simulink model "physical_model"  (R2016b)
settings: Solver=VariableStepAuto  StartTime=0.0  StopTime=3000  FixedStep=1  RelTol=1e-3  AbsTol=1e-6
model workspace (MATLAB code in the model file):
  | % load initial conditions and physical properties from file
  | 
  | %sldemo_househeat_data
  | househeat_data_szakdoga
  | 
  | addpath('subsystems')
  | 
  | %disp('adding models...')
  | load('subsystems/mpc_floor_radiator.mat')
  | %disp('done.')
values from neighbouring files (symbols this model uses):
  A_heater = 3.5    [househeat_data_szakdoga.m]
  c = 1005.4    [househeat_data_szakdoga.m]
  h_heater = 11    [househeat_data_szakdoga.m]
  M = (lenHouse*widHouse*htHouse+tan(pitRoof)*widHouse*lenHouse)*densAir    [househeat_data_szakdoga.m]    (also in thesismpcmiso.m = A1\L)
  Req = RWall*RWindow/(RWall + RWindow)    [househeat_data_szakdoga.m]
  supp_water_initial_temp = 0    [househeat_data_szakdoga.m]
  TinHeatK = 273    [househeat_data_szakdoga.m]
  TinIC = 0    [househeat_data_szakdoga.m]
undefined symbols (not defined in the file or in its folder): timeUnit_1hour, timeUnit_1min, timeUnit_1week
libraries: fl_lib x37, nesl_utility x14, simulink x3, instrumentlib x3, xpcrtudplib x3, slident x1, mpclib x1
Description:
  | Thermal Model of a House
  | 
  | This demo illustrates how you can use Simulink(R) to create the thermal model of
  | a house. This system models the outdoor environment, the thermal
  | characteristics of the house, and the house heating system.
  | 
  | The sldemo_househeat_data.m file initializes data in the model workspace.
  | To make changes, you can edit the model workspace directly or edit the MATLAB(R) file
  | and re-load the model workspace.
  | 
  | To view the model workspace, select View > Model Explorer
  | from the Simulink editor.
  | 
  | Note: Time is given in units of hours
settings Model: PauseTimes=10  ExtModeTrigMode=oneshot  ExtModeArmWhenConnect=off  ExtModeAutoUpdateStatusClock=off  Creator=The MathWorks, Inc.  LastModifiedBy=gylaszlo
settings DataIOCC: ExternalInput=[]  InitialState=[]  SaveFormat=StructureWithTime  SaveOutput=off  SaveTime=off  SignalLoggingName=sldemo_househeat_output
settings OptimizationCC: BlockReduction=off  BooleanDataType=off  ExpressionDepthLimit=2147483647  InitFltsAndDblsToZero=on  LifeSpan=inf  BufferReusableBoundary=off
settings DebuggingCC: SaveWithParameterizedLinksMsg=none  UnderspecifiedInitializationDetection=Classic  MergeDetectMultiDrivingBlocksExec=none  SignalResolutionControl=TryResolveAllWithWarning  MultiTaskDSMMsg=warning  MultiTaskCondExecSysMsg=none  IntegerOverflowMsg=none  FcnCallInpInsideContextMsg=warning  BusObjectLabelMismatch=none  StateNameClashWarn=warning  SFUnexpectedBacktrackingDiag=warning  SFNoUnconditionalDefaultTransitionDiag=warning  SFExecutionAtInitializationDiag=none  IntegerSaturationMsg=none
settings HardwareCC: ProdBitPerPointer=32  ProdBitPerSizeT=32  ProdBitPerPtrDiffT=32  ProdLargestAtomicFloat=None  ProdIntDivRoundTo=Undefined  ProdEndianess=Unspecified  ProdWordSize=32  ProdHWDeviceType=32-bit Generic  TargetUnknown=on
settings ModelReferenceCC: PropagateSignalLabelsOutOfModel=off
settings GRTTargetCC: TargetFcnLib=ansi_tfl_tmw.mat  TargetLangStandard=C89/C90 (ANSI)  GeneratePreprocessorConditionals=Disable all  CombineOutputUpdateFcns=off  GRTInterface=on
settings ConfigComp: CovMetricSettings=dw  CovHtmlReporting=on  CovSaveCumulativeToWorkspaceVar=on  CovSaveSingleToWorkspaceVar=on  CovExternalEMLEnable=off

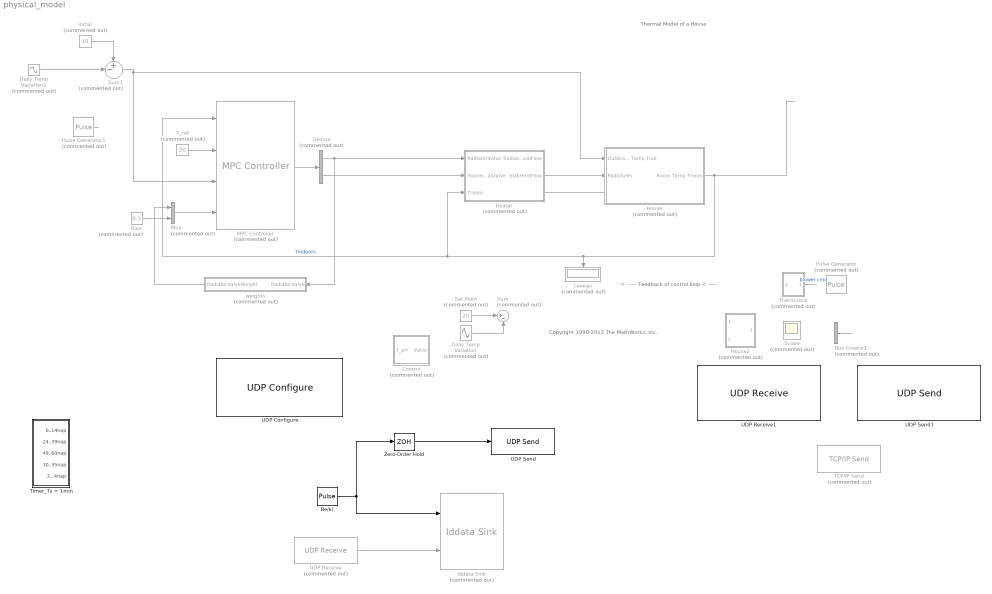
== system physical_model ==
  note: < ------ Feedback of control loop < ------
  note: Thermal Model of a House
  note: Copyright 1990-2012 The MathWorks, Inc.
  Be/ki : DiscretePulseGenerator  PulseType=Time based  Amplitude=100  Period=120  PulseWidth=50
  Bus Creator1 : BusCreator  Commented=on  Inputs=2
  Control : Subsystem  Commented=on
  Daily Temp Variation : Sin  Commented=on  Amplitude=5  Frequency=3.14*2/3600/24  Phase=3.14/2  SampleTime=0
  Daily Temp Variation1 : Sin  Commented=on  Amplitude=5  Frequency=3.14*2/3600/24  Phase=3.14/2  SampleTime=0
  Demux : Demux  Commented=on  Outputs=2
  Heater : Subsystem  Commented=on
  House : Subsystem  Commented=on
  House2 : Subsystem  Commented=on
      mask Display: image(fullfile(matlabroot,'toolbox','simulink','simdemos','simgeneral','images','HouseHeatHousePix.svg'))
  Iddata Sink : slident/Iddata Sink  Commented=on  datasetname=meres  Ts=10  isu=off  isy=off
  Levego : Display  Commented=on
  MPC Controller : mpclib/MPC Controller  Commented=on  SCDEnableBlockLinearizationSpecification=on  mpcobj=mpc_floor_radiator  is_multiple=0  enable_value=0  return_u0=off  ref_from_ws=off  ref_signal_name=[]  ref_preview=off  md_from_ws=off  md_signal_name=[]  md_preview=off  from_project=off  project_file=MPCtask.mat  md_inport=on  mv_inport=off  cost_outport=off  return_sequence=off  return_qpstatus=off  return_state=off  state_inport=off  lims_inport=off  ywt_inport=off  is_designfromscratch=0  uwt_inport=on  duwt_inport=off  rhoeps_inport=off  uref_inport=off  n_ts=300  n_mv=2  n_md=1  n_ud=0  n_mo=1  n_uo=0  BlockDataType=double  SampleTimeInherited=off  switch_inport=off
  Mux : Mux  Commented=on  Inputs=2
  Pulse Generator : DiscretePulseGenerator  Commented=on  PulseType=Time based  Period=3600*24*4  PulseWidth=50
  Pulse Generator1 : DiscretePulseGenerator  Commented=on  PulseType=Time based  Amplitude=15  Period=3600*24*4  PulseWidth=50
  Scope : Scope  Commented=on
  Set Point : Constant  Commented=on  Value=20
  Sum : Sum  Commented=on  Inputs=+-|  SaturateOnIntegerOverflow=on  InputSameDT=on  OutDataTypeStr=Inherit: Same as first input
  Sum1 : Sum  Commented=on  Inputs=+-|  SaturateOnIntegerOverflow=on  InputSameDT=on  OutDataTypeStr=Inherit: Same as first input
  TCP/IP Send : instrumentlib/TCP//IP Send  Commented=on  Host=192.168.0.108  Port=9090  EnableBlockingMode=on  Timeout=10  ByteOrder=BigEndian
  T_ref : Constant  Commented=on  Value=20
  Thermostat : Subsystem  Commented=on
      mask Display: image(fullfile(matlabroot,'toolbox','simulink','simdemos','simgeneral','images','HouseHeatThermostatPix.svg'))
  Timer_Ts = 1min : Subsystem
  UDP Configure : xpcrtudplib/UDP Configure  Priority=-1  IpAddress=192.168.0.136  SubnetMask=255.255.255.0  Gateway=192.168.0.1  PciBus=2  PciSlot=0  ID=1  tune=0
  UDP Receive : instrumentlib/UDP Receive  Commented=on  Port=9090  LocalPort=-1  DataSize=[1 1]  EnableBlockingMode=on  Timeout=10  SampleTime=0.01  DataType=uint8  ByteOrder=BigEndian
  UDP Receive1 : xpcrtudplib/UDP Receive  ipAddressVal=Use host-target connection  localPort=8001  rcvWidth=16  rcvFmAny=on  fmAddress=0.0.0.0  sampleTime=-1
  UDP Send : instrumentlib/UDP Send  Host=192.168.0.108  Port=9090  LocalPort=-1  EnableBlockingMode=on  ByteOrder=BigEndian
  UDP Send1 : xpcrtudplib/UDP Send  ipAddressVal=Use host-target connection  localPort=9090  toAddress=168.192.0.108  toPort=9090  sampleTime=-1
  Zero-Order Hold : ZeroOrderHold  SampleTime=10
  floor : Constant  Commented=on  Value=0.3
  initial : Constant  Commented=on  Value=10
  weights : Subsystem  Commented=on
  wires:
  ? -> Control/1(T_err)  "Terr"
  House/1(Room Temp Troom) -> Heater/3(Troom), MPC Controller/1, Levego/1  "Tindoors"
  Set Point/1 -> Sum/1
  Thermostat/1(Blower switch) -> ?  "blower cmd"
  Bus Creator1/1 -> ?
  Sum1/1 -> MPC Controller/3, House/1(Outdoor Temp Tout)
  Daily Temp Variation/1 -> Sum/2
  T_ref/1 -> MPC Controller/2
  Heater/2(SlabHeatFlow) -> House/2(Padlofutes)
  Daily Temp Variation1/1 -> Sum1/2
  initial/1 -> Sum1/1
  MPC Controller/1 -> Demux/1
  Demux/2 -> Heater/2(FloorHeatValve)
  Demux/1 -> weights/1(RadiatorValve), Heater/1(RadiatorValve)
  Pulse Generator1/1 -> ?
  weights/1(RadiatorValveWeight) -> Mux/1
  floor/1 -> Mux/2
  Mux/1 -> MPC Controller/4
  UDP Receive/1 -> Iddata Sink/2
  Be/ki/1 -> Zero-Order Hold/1, Iddata Sink/1
  Zero-Order Hold/1 -> UDP Send/1
  connections:
  House/LConn1 -- Heater/RConn1

== system physical_model/Control ==
  note: valve opening rate
  T_err : Inport
  PID Controller : simulink/Continuous/PID Controller  Controller=PI  TimeDomain=Continuous-time  SampleTime=-1  IntegratorMethod=Forward Euler  FilterMethod=Forward Euler  Form=Parallel  UseFilter=on  ControllerParametersSource=internal  P=0.09  I=9.95e-07  D=0  N=100  InitialConditionSource=internal  InitialConditionForIntegrator=0  InitialConditionForFilter=0  ExternalReset=none  LimitOutput=on  UpperSaturationLimit=1  LowerSaturationLimit=0  LinearizeAsGain=on  AntiWindupMode=none  Kb=1  TrackingMode=off  Kt=1  PParamMin=[]  PParamMax=[]  IParamMin=[]  IParamMax=[]  DParamMin=[]  DParamMax=[]  NParamMin=[]  NParamMax=[]  KbParamMin=[]  KbParamMax=[]  KtParamMin=[]  KtParamMax=[]  POutMin=[]  POutMax=[]  IOutMin=[]  IOutMax=[]  DOutMin=[]  DOutMax=[]  NOutMin=[]  NOutMax=[]  KbOutMin=[]  KbOutMax=[]  KtOutMin=[]  KtOutMax=[]  IntegratorOutMin=[]  IntegratorOutMax=[]  FilterOutMin=[]  FilterOutMax=[]  SumOutMin=[]  SumOutMax=[]  SumI1OutMin=[]  SumI1OutMax=[]  SumI2OutMin=[]  SumI2OutMax=[]  SumI3OutMin=[]  SumI3OutMax=[]  SumDOutMin=[]  SumDOutMax=[]  SaturationOutMin=[]  SaturationOutMax=[]  IntegratorContinuousStateAttributes=''  IntegratorStateMustResolveToSignalObject=off  IntegratorRTWStateStorageClass=Auto  FilterContinuousStateAttributes=''  FilterStateMustResolveToSignalObject=off  FilterRTWStateStorageClass=Auto  DifferentiatorICPrevScaledInput=0  DifferentiatorOutMin=[]  DifferentiatorOutMax=[]
  Valve : Outport
  wires:
  T_err/1 -> PID Controller/1
  PID Controller/1 -> Valve/1

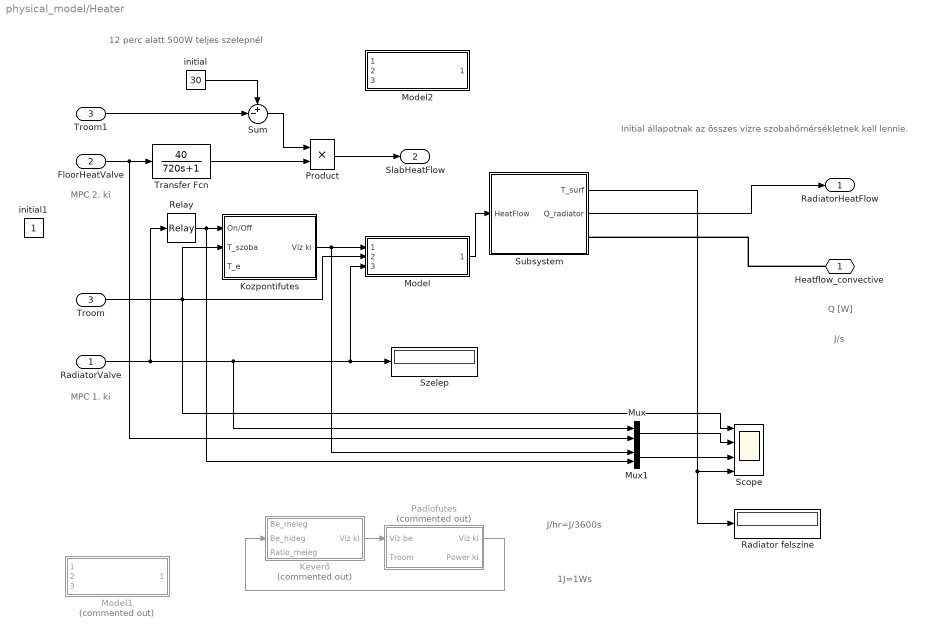
== system physical_model/Heater ==
  note: MPC 1. ki
  note: 12 perc alatt 500W teljes szelepnél
  note: Initial állapotnak az összes vízre szobahőmérsékletnek kell lennie.
  note: J/s
  note: 1J=1Ws
  note: J/hr=J/3600s
  note: Q [W]
  note: MPC 2. ki
  RadiatorValve : Inport
  FloorHeatValve : Inport  Port=2
  Troom : Inport  Port=3
  Keverő : Subsystem  Commented=on
  Kozpontifutes : Subsystem
  Model : ModelReference  ModelNameDialog=Radiator  SimulationMode=Normal  ModelReferenceVersion=1.21
  Model1 : ModelReference  Commented=on  ModelNameDialog=Radiator  SimulationMode=Normal  ModelReferenceVersion=1.21
  Model2 : ModelReference  ModelNameDialog=Radiator  SimulationMode=Normal  ModelReferenceVersion=1.21
  Mux : Mux  Inputs=2
  Mux1 : Mux  Inputs=2
  Padlofutes : Subsystem  Commented=on
  Product : Product
  Radiator felszine : Display
  Relay : Relay
  Scope : Scope  NumInputPorts=4
  Subsystem : Subsystem
  Sum : Sum  Inputs=+-|
  Szelep : Display
  Transfer Fcn : TransferFcn  Numerator=[40]  Denominator=[720 1]
  Troom1 : InportShadow  Port=3
  initial : Constant  Value=30
  initial1 : Constant
  Heatflow_convective : PMIOPort  Port=1  Side=Right
  RadiatorHeatFlow : Outport
  SlabHeatFlow : Outport  Port=2
  wires:
  Troom/1 -> Scope/1, Model/2, Kozpontifutes/2(T_szoba)
  Kozpontifutes/1(Víz ki) -> Mux1/1, Model/1
  ? -> ?
  Padlofutes/1(Víz ki) -> Keverő/2(Be_hideg)
  Subsystem/1(T_surf) -> Scope/4, Radiator felszine/1
  Keverő/1(Víz ki) -> Padlofutes/1(Víz be)
  RadiatorValve/1 -> Relay/1, Mux/1, Szelep/1, Model/3
  Model/1 -> Subsystem/1(HeatFlow)
  FloorHeatValve/1 -> Mux/2, Transfer Fcn/1
  Subsystem/2(Q_radiator) -> RadiatorHeatFlow/1
  Troom1/1 -> Sum/2
  Product/1 -> SlabHeatFlow/1
  Transfer Fcn/1 -> Product/2
  Sum/1 -> Product/1
  initial/1 -> Sum/1
  Mux/1 -> Scope/2
  Relay/1 -> Mux1/2, Kozpontifutes/1(On/Off)
  Mux1/1 -> Scope/3
  connections:
  Heatflow_convective/RConn1 -- Subsystem/RConn1

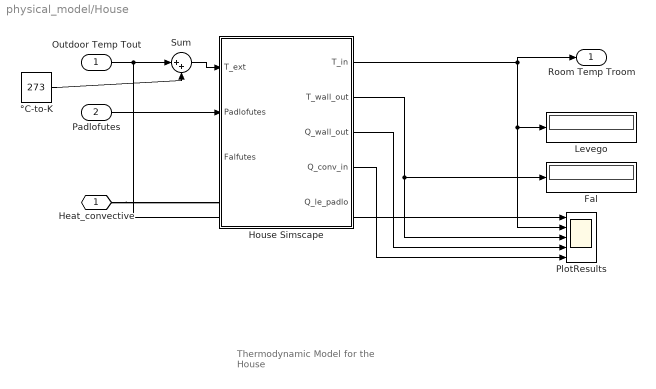
== system physical_model/House ==
  note: Thermodynamic Model
      | for the House
  Outdoor Temp Tout : Inport
  Padlofutes : Inport  Port=2
  Fal : Display
  House Simscape : Subsystem
  Levego : Display
  PlotResults : Scope  NumInputPorts=5
  Sum : Sum  Inputs=|++
  °C-to-K : Constant  Value=273
  Heat_convective : PMIOPort  Port=1  Side=Left
  Room Temp Troom : Outport  InitialOutput=0
  wires:
  Outdoor Temp Tout/1 -> Sum/1, PlotResults/1
  House Simscape/3(Q_wall_out) -> PlotResults/4
  Sum/1 -> House Simscape/1(T_ext)
  °C-to-K/1 -> Sum/2
  House Simscape/1(T_in) -> Room Temp Troom/1, PlotResults/2, Levego/1
  House Simscape/2(T_wall_out) -> Fal/1, PlotResults/3
  House Simscape/4(Q_conv_in) -> PlotResults/5
  Padlofutes/1 -> House Simscape/2(Padlofutes)
  connections:
  Heat_convective/RConn1 -- House Simscape/LConn1

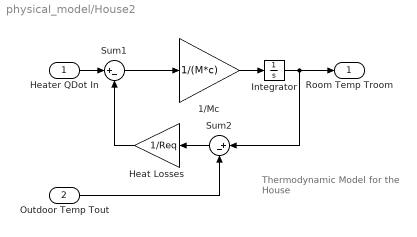
== system physical_model/House2 ==
  note: Thermodynamic Model
      | for the House
  Heater QDot In : Inport
  Outdoor Temp Tout : Inport  Port=2
  1/Mc : Gain  Gain=1/(M*c)  SaturateOnIntegerOverflow=on  OutDataTypeStr=Inherit: Same as input  ParamDataTypeStr=Inherit: Same as input
  Heat Losses : Gain  Gain=1/Req  SaturateOnIntegerOverflow=on  OutDataTypeStr=Inherit: Same as input  ParamDataTypeStr=Inherit: Same as input
  Integrator : Integrator  InitialCondition=TinIC
  Sum1 : Sum  Inputs=|+-  SaturateOnIntegerOverflow=on  InputSameDT=on  OutDataTypeStr=Inherit: Same as first input
  Sum2 : Sum  Inputs=|+-  SaturateOnIntegerOverflow=on  InputSameDT=on  OutDataTypeStr=Inherit: Same as first input
  Room Temp Troom : Outport  InitialOutput=0
  wires:
  Outdoor Temp Tout/1 -> Sum2/2
  Heater QDot In/1 -> Sum1/1
  Sum1/1 -> 1/Mc/1
  Sum2/1 -> Heat Losses/1
  Heat Losses/1 -> Sum1/2
  1/Mc/1 -> Integrator/1
  Integrator/1 -> Sum2/1, Room Temp Troom/1

== system physical_model/Thermostat ==
  note: Thermostat Subsystem
  Terr : Inport
  Relay1 : Relay  OnSwitchValue=1  OffSwitchValue=-1
  Blower switch : Outport  InitialOutput=0
  wires:
  Terr/1 -> Relay1/1
  Relay1/1 -> Blower switch/1

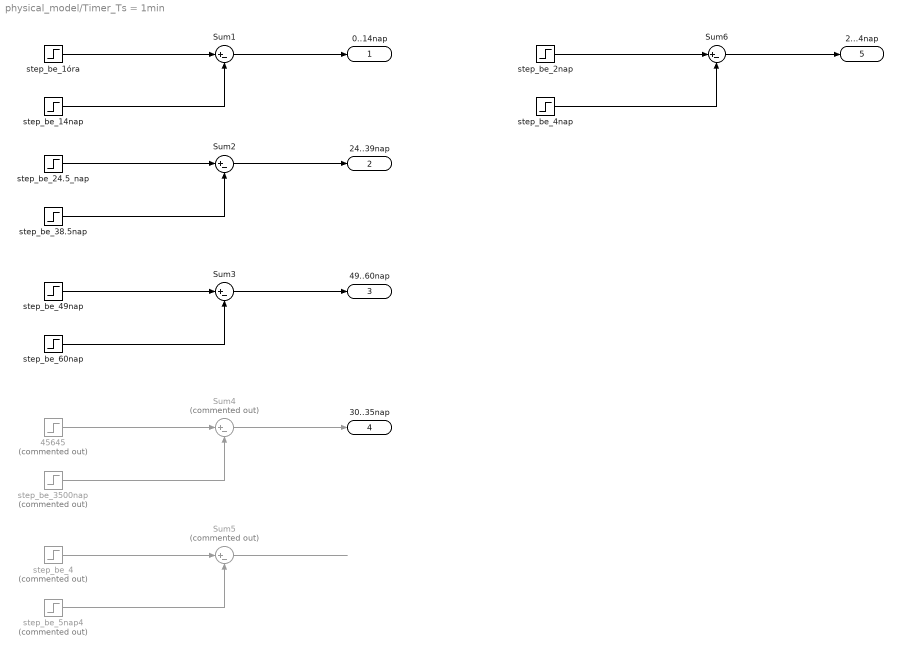
== system physical_model/Timer_Ts = 1min ==
  45645 : Step  Commented=on  Time=3600*24*30  SampleTime=0
  Sum{1..3,6} (4 alike) : Sum  Inputs=|+-  SaturateOnIntegerOverflow=on  InputSameDT=on  OutDataTypeStr=Inherit: Same as first input
  Sum4 : Sum  Commented=on  Inputs=|+-  SaturateOnIntegerOverflow=on  InputSameDT=on  OutDataTypeStr=Inherit: Same as first input
  Sum5 : Sum  Commented=on  Inputs=|+-  SaturateOnIntegerOverflow=on  InputSameDT=on  OutDataTypeStr=Inherit: Same as first input
  step_be_14nap : Step  Time=timeUnit_1week*2  SampleTime=0
  step_be_1óra : Step  Time=timeUnit_1hour  SampleTime=0
  step_be_24.5_nap : Step  Time=timeUnit_1week*3.5  SampleTime=0
  step_be_2nap : Step  Time=3600*24*2  SampleTime=0
  step_be_3500nap : Step  Commented=on  Time=3600*24*35  SampleTime=0
  step_be_38.5nap : Step  Time=timeUnit_1week*5.5  SampleTime=0
  step_be_4 : Step  Commented=on  Time=0  SampleTime=0
  step_be_49nap : Step  Time=timeUnit_1week*7  SampleTime=0
  step_be_4nap : Step  Time=3600*24*4  SampleTime=0
  step_be_5nap4 : Step  Commented=on  Time=3600*24*5  SampleTime=0
  step_be_60nap : Step  Time=timeUnit_1week*9  SampleTime=0
  0..14nap : Outport
  24..39nap : Outport  Port=2
  49..60nap : Outport  Port=3
  30..35nap : Outport  Port=4
  2...4nap : Outport  Port=5
  wires:
  Sum1/1 -> 0..14nap/1
  step_be_14nap/1 -> Sum1/2
  step_be_1óra/1 -> Sum1/1
  Sum2/1 -> 24..39nap/1
  step_be_38.5nap/1 -> Sum2/2
  step_be_24.5_nap/1 -> Sum2/1
  Sum3/1 -> 49..60nap/1
  step_be_60nap/1 -> Sum3/2
  step_be_49nap/1 -> Sum3/1
  Sum4/1 -> 30..35nap/1
  step_be_3500nap/1 -> Sum4/2
  45645/1 -> Sum4/1
  Sum5/1 -> ?
  step_be_5nap4/1 -> Sum5/2
  step_be_4/1 -> Sum5/1
  Sum6/1 -> 2...4nap/1
  step_be_4nap/1 -> Sum6/2
  step_be_2nap/1 -> Sum6/1

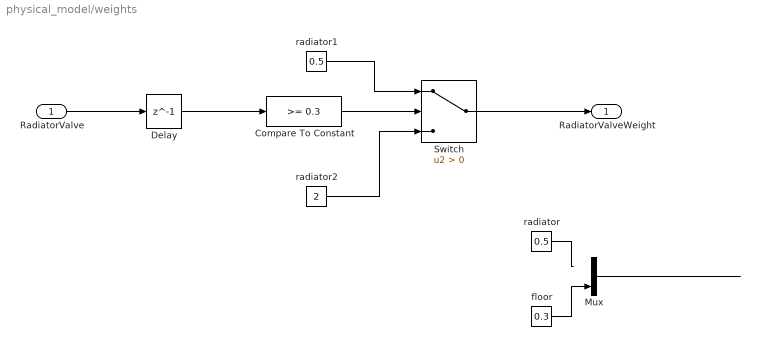
== system physical_model/weights ==
  RadiatorValve : Inport
  Compare To Constant : simulink/Logic and Bit Operations/Compare To Constant  relop=>=  const=0.3  OutDataTypeStr=boolean
  Delay : Delay  DelayLength=1  InitialCondition=0
  Mux : Mux  Inputs=2
  Switch : Switch  Criteria=u2 > Threshold
  floor : Constant  Value=0.3
  radiator : Constant  Value=0.5
  radiator1 : Constant  Value=0.5
  radiator2 : Constant  Value=2
  RadiatorValveWeight : Outport
  wires:
  Mux/1 -> ?
  radiator/1 -> ?
  floor/1 -> Mux/2
  Compare To Constant/1 -> Switch/2
  radiator1/1 -> Switch/1
  radiator2/1 -> Switch/3
  Switch/1 -> RadiatorValveWeight/1
  RadiatorValve/1 -> Delay/1
  Delay/1 -> Compare To Constant/1

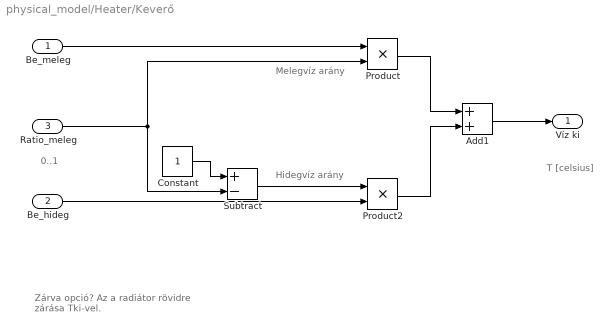
== system physical_model/Heater/Keverő ==
  note: T [celsius]
  note: Hidegvíz arány
  note: Zárva opció?
      | Az a radiátor rövidre zárása Tki-vel.
  note: 0..1
  note: Melegvíz arány
  Be_meleg : Inport
  Be_hideg : Inport  Port=2
  Ratio_meleg : Inport  Port=3
  Add1 : Sum
  Constant : Constant
  Product : Product
  Product2 : Product
  Subtract : Sum  Inputs=+-
  Víz ki : Outport
  wires:
  Be_meleg/1 -> Product/1
  Ratio_meleg/1 -> Subtract/2, Product/2
  Constant/1 -> Subtract/1
  Be_hideg/1 -> Product2/2
  Subtract/1 -> Product2/1
  Product/1 -> Add1/1
  Product2/1 -> Add1/2
  Add1/1 -> Víz ki/1

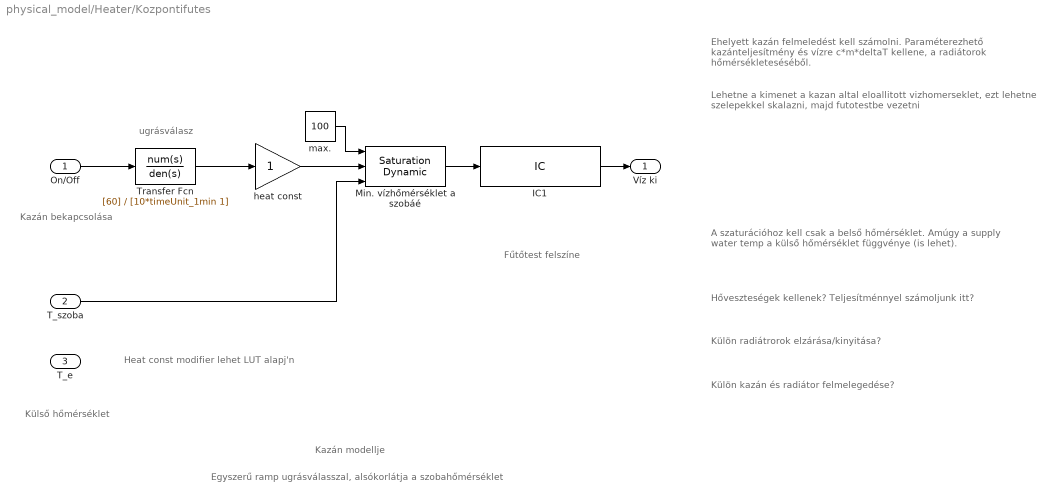
== system physical_model/Heater/Kozpontifutes ==
  note: Egyszerű ramp ugrásválasszal, alsókorlátja a szobahőmérséklet
  note: Kazán modellje
  note: Heat const modifier lehet LUT alapj'n
  note: Hőveszteségek kellenek? Teljesítménnyel számoljunk itt?
  note: Ehelyett kazán felmeledést kell számolni. Paraméterezhető kazánteljesítmény és vízre c*m*deltaT kellene, a radiátorok hőmérsékleteséséből.
  note: A szaturációhoz kell csak a belső hőmérséklet. Amúgy a supply water temp a külső hőmérséklet függvénye (is lehet).
  note: Lehetne a kimenet a kazan altal eloallitott vizhomerseklet, ezt lehetne szelepekkel skalazni, majd futotestbe vezetni
  note: Külön kazán és radiátor felmelegedése?
  note: Külön radiátrorok elzárása/kinyitása?
  note: ugrásválasz
  note: Külső hőmérséklet
  note: Kazán bekapcsolása
  note: Fűtőtest felszíne
  On/Off : Inport
  T_szoba : Inport  Port=2
  T_e : Inport  Port=3
  IC1 : InitialCondition  Value=supp_water_initial_temp
  Min. vízhőmérséklet a szobáé : simulink/Discontinuities/Saturation Dynamic  OutMin=[]  OutMax=[]  OutDataTypeStr=Inherit: Same as second input  OutDataType=fixdt(1, 16)  OutScaling=2^-10  DoSatur=off
  Transfer Fcn : TransferFcn  Numerator=[60]  Denominator=[10*timeUnit_1min 1]
  heat const : Gain
  max. : Constant  Value=100
  Víz ki : Outport
  wires:
  max./1 -> Min. vízhőmérséklet a szobáé/1
  Min. vízhőmérséklet a szobáé/1 -> IC1/1
  T_szoba/1 -> Min. vízhőmérséklet a szobáé/3
  heat const/1 -> Min. vízhőmérséklet a szobáé/2
  On/Off/1 -> Transfer Fcn/1
  Transfer Fcn/1 -> heat const/1
  IC1/1 -> Víz ki/1

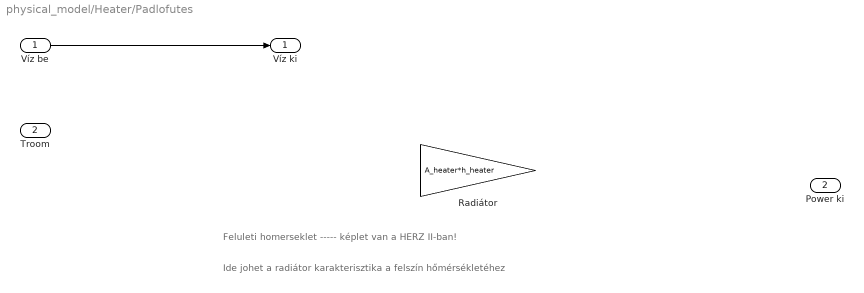
== system physical_model/Heater/Padlofutes ==
  note: Ide johet a radiátor karakterisztika a felszín hőmérsékletéhez
  note: Feluleti homerseklet ----- képlet van a HERZ II-ban!
  Víz be : Inport
  Troom : Inport  Port=2
  Radiátor : Gain  Gain=A_heater*h_heater
  Víz ki : Outport
  Power ki : Outport  Port=2
  wires:
  Víz be/1 -> Víz ki/1

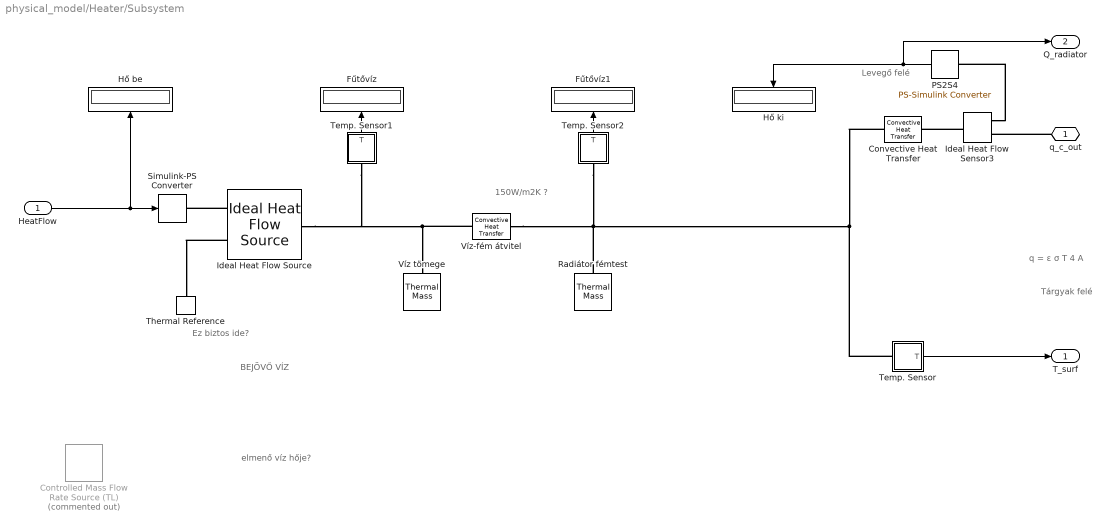
== system physical_model/Heater/Subsystem ==
  note: elmenő víz hője?
  note: BEJÖVŐ VÍZ
  note: q = ε σ T 4 A
  note: 150W/m2K ?
  note: Tárgyak felé
  note: Levegő felé
  note: Ez biztos ide?
  HeatFlow : Inport
  Controlled Mass Flow Rate Source (TL) : fl_lib/Thermal Liquid/Sources/Controlled Mass Flow Rate Source (TL)  Commented=on  area=0.01 m^2  length=0.1 m
  Convective Heat Transfer : fl_lib/Thermal/Thermal Elements/Convective Heat Transfer  area=area_radiator m^2  heat_tr_coeff=h_c_radi W/(m^2 * K)  Q_specify=off  Q_priority=None  Q=0 J/s  T_specify=off  T_priority=None  T=0 K
  Fűtővíz : Display
  Fűtővíz1 : Display
  Hő be : Display
  Hő ki : Display
  Ideal Heat Flow Sensor3 : fl_lib/Thermal/Thermal Sensors/Ideal Heat Flow Sensor
  Ideal Heat Flow Source : fl_lib/Thermal/Thermal Sources/Ideal Heat Flow Source
  PS2S4 : nesl_utility/PS-Simulink Converter  PhysicalDomain=network_engine_domain  SubClassName=ps_output  LeftPortType=input  RightPortType=output  PseudoPeriodic=off  Frequencies=[]  Unit=J/s  AffineConversion=on
  Radiátor fémtest : fl_lib/Thermal/Thermal Elements/Thermal Mass  mass=m_r kg  sp_heat=c_metal J/kg/K  T_specify=on  T_priority=High  T=TinHeatK K  Q_specify=off  Q_priority=None  Q=0 J/s
  Simulink-PS Converter : nesl_utility/Simulink-PS Converter  PhysicalDomain=network_engine_domain  SubClassName=ps_input  LeftPortType=input  RightPortType=output  PseudoPeriodic=off  Frequencies=[]  NoiseDistribution=none  NoiseParameters=[]  Unit=1  AffineConversion=off  InputFiltering=off  SimscapeFilterOrder=1  InputFilterTimeConstant=0.001  UdotUserProvided=1
  Temp. Sensor : Subsystem
  Temp. Sensor1 : Subsystem
  Temp. Sensor2 : Subsystem
  Thermal Reference : fl_lib/Thermal/Thermal Elements/Thermal Reference
  Víz tömege : fl_lib/Thermal/Thermal Elements/Thermal Mass  mass=m_w_r kg  sp_heat=c_w J/kg/K  T_specify=on  T_priority=High  T=TinHeatK K  Q_specify=off  Q_priority=None  Q=0 J/s
  Víz-fém átvitel : fl_lib/Thermal/Thermal Elements/Convective Heat Transfer  area=area_radiator m^2  heat_tr_coeff=h_w_radi W/(m^2 * K)  Q_specify=off  Q_priority=None  Q=0 J/s  T_specify=off  T_priority=None  T=0 K
  q_c_out : PMIOPort  Port=1  Side=Right
  T_surf : Outport
  Q_radiator : Outport  Port=2
  wires:
  HeatFlow/1 -> Hő be/1, Simulink-PS Converter/1
  Temp. Sensor/1(T) -> T_surf/1
  Temp. Sensor1/1(T) -> Fűtővíz/1
  Temp. Sensor2/1(T) -> Fűtővíz1/1
  PS2S4/1 -> Q_radiator/1, Hő ki/1
  connections:
  Ideal Heat Flow Source/RConn1 -- Simulink-PS Converter/RConn1
  Radiátor fémtest/LConn1 -- Convective Heat Transfer/LConn1 -- Temp. Sensor/LConn1 -- Temp. Sensor2/LConn1 -- Víz-fém átvitel/RConn1
  Víz-fém átvitel/LConn1 -- Ideal Heat Flow Source/LConn1 -- Temp. Sensor1/LConn1 -- Víz tömege/LConn1
  Ideal Heat Flow Source/RConn2 -- Thermal Reference/LConn1
  Ideal Heat Flow Sensor3/RConn1 -- PS2S4/LConn1
  q_c_out/RConn1 -- Ideal Heat Flow Sensor3/RConn2
  Ideal Heat Flow Sensor3/LConn1 -- Convective Heat Transfer/RConn1

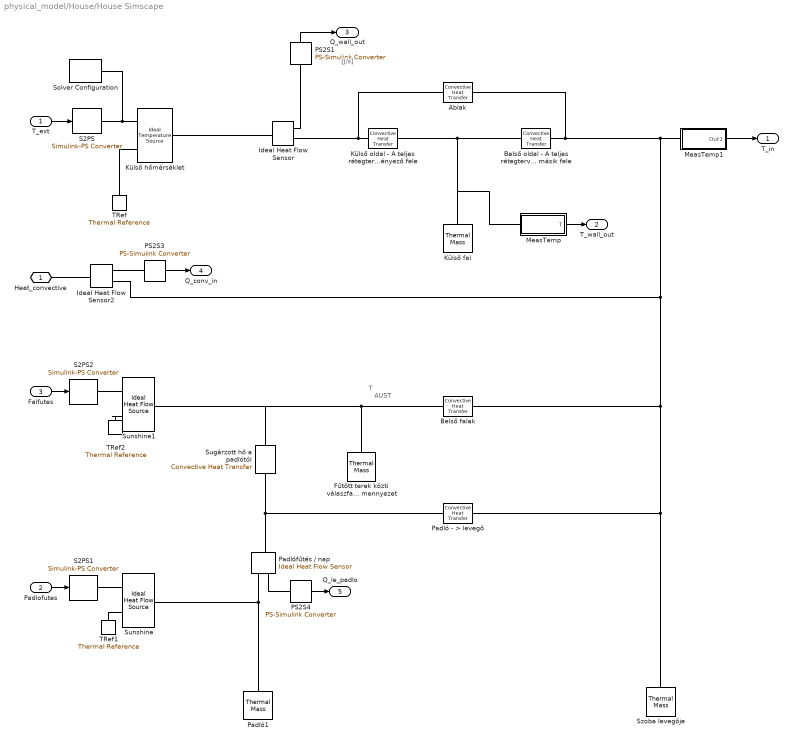
== system physical_model/House/House Simscape ==
  note: T
  note: AUST
  note: [J/s]
  T_ext : Inport
  Padlofutes : Inport  Port=2
  Falfutes : Inport  Port=3
  Ablak : fl_lib/Thermal/Thermal Elements/Convective Heat Transfer  area=4 m^2  heat_tr_coeff=4 W/(m^2 * K)  Q_specify=off  Q_priority=None  Q=0 J/s  T_specify=off  T_priority=None  T=0 K
  Belső falak : fl_lib/Thermal/Thermal Elements/Convective Heat Transfer  area=65 m^2  heat_tr_coeff=7 W/(m^2 * K)  Q_specify=off  Q_priority=None  Q=0 J/s  T_specify=off  T_priority=None  T=0 K
  Belső oldal - A teljes rétegtervi hőátbocsátási tényező másik fele : fl_lib/Thermal/Thermal Elements/Convective Heat Transfer  area=4.5 m^2  heat_tr_coeff=8 W/(m^2 * K)  Q_specify=off  Q_priority=None  Q=0 J/s  T_specify=off  T_priority=None  T=0 K
  "Fűtött terek közti válaszfalak, mennyezet" : fl_lib/Thermal/Thermal Elements/Thermal Mass  mass=6000 kg  sp_heat=840 J/kg/K  T_specify=on  T_priority=High  T=TinIC degC  Q_specify=off  Q_priority=None  Q=0 J/s
      settings: LogSimulationData=on
  Ideal Heat Flow Sensor : fl_lib/Thermal/Thermal Sensors/Ideal Heat Flow Sensor
  Ideal Heat Flow Sensor2 : fl_lib/Thermal/Thermal Sensors/Ideal Heat Flow Sensor
  Külső fal : fl_lib/Thermal/Thermal Elements/Thermal Mass  mass=1200 kg  sp_heat=840 J/kg/K  T_specify=on  T_priority=High  T=TinIC degC  Q_specify=off  Q_priority=None  Q=0 J/s
      settings: LogSimulationData=on
  Külső hőmérséklet : fl_lib/Thermal/Thermal Sources/Ideal Temperature Source
  Külső oldal - A teljes rétegtervi hőátbocsátási tényező fele : fl_lib/Thermal/Thermal Elements/Convective Heat Transfer  area=4.5 m^2  heat_tr_coeff=0.6 W/(m^2 * K)  Q_specify=off  Q_priority=None  Q=0 J/s  T_specify=off  T_priority=None  T=0 K
  MeasTemp : Subsystem
  MeasTemp1 : Subsystem
  PS2S1 : nesl_utility/PS-Simulink Converter  PhysicalDomain=network_engine_domain  SubClassName=ps_output  LeftPortType=input  RightPortType=output  PseudoPeriodic=off  Frequencies=[]  Unit=J/s  AffineConversion=on
  PS2S3 : nesl_utility/PS-Simulink Converter  PhysicalDomain=network_engine_domain  SubClassName=ps_output  LeftPortType=input  RightPortType=output  PseudoPeriodic=off  Frequencies=[]  Unit=J/s  AffineConversion=on
  PS2S4 : nesl_utility/PS-Simulink Converter  PhysicalDomain=network_engine_domain  SubClassName=ps_output  LeftPortType=input  RightPortType=output  PseudoPeriodic=off  Frequencies=[]  Unit=J/s  AffineConversion=on
  Padló - > levegő : fl_lib/Thermal/Thermal Elements/Convective Heat Transfer  area=16 m^2  heat_tr_coeff=4 W/(m^2 * K)  Q_specify=off  Q_priority=None  Q=0 J/s  T_specify=off  T_priority=None  T=0 K
  Padló1 : fl_lib/Thermal/Thermal Elements/Thermal Mass  mass=2000 kg  sp_heat=840 J/kg/K  T_specify=on  T_priority=High  T=TinIC degC  Q_specify=off  Q_priority=None  Q=0 J/s
      settings: LogSimulationData=on
  Padlófűtés / nap : fl_lib/Thermal/Thermal Sensors/Ideal Heat Flow Sensor
  S2PS : nesl_utility/Simulink-PS Converter  PhysicalDomain=network_engine_domain  SubClassName=ps_input  LeftPortType=input  RightPortType=output  PseudoPeriodic=off  Frequencies=[]  NoiseDistribution=none  NoiseParameters=[]  Unit=1  AffineConversion=off  InputFiltering=off  SimscapeFilterOrder=1  InputFilterTimeConstant=.001  UdotUserProvided=0
  S2PS1 : nesl_utility/Simulink-PS Converter  PhysicalDomain=network_engine_domain  SubClassName=ps_input  LeftPortType=input  RightPortType=output  PseudoPeriodic=off  Frequencies=[]  NoiseDistribution=none  NoiseParameters=[]  Unit=1  AffineConversion=off  InputFiltering=off  SimscapeFilterOrder=1  InputFilterTimeConstant=.001  UdotUserProvided=0
  S2PS2 : nesl_utility/Simulink-PS Converter  PhysicalDomain=network_engine_domain  SubClassName=ps_input  LeftPortType=input  RightPortType=output  PseudoPeriodic=off  Frequencies=[]  NoiseDistribution=none  NoiseParameters=[]  Unit=1  AffineConversion=off  InputFiltering=off  SimscapeFilterOrder=1  InputFilterTimeConstant=.001  UdotUserProvided=0
  Solver Configuration : nesl_utility/Solver Configuration  PhysicalDomain=network_engine_domain  SubClassName=solver  LeftPortType=input  RightPortType=generic  Accelerate=off  Tones=[]  Harmonics=[]  SimulateNoise=off  Profile=off  UseLocalSampling=off  EnableSwitchedLinearOptims=on  FrequencyDomain=off  UseCCode=off  RelTol=0.001  AbsTol=1e-06  MinStep=1e-09  ToWorkspace=off  RevertToSquareIcSolve=off  NumHomotopyIterations=100  PhasorMode=off  PhasorModeNumHarmonics=1  OverrideAbsTol=off  DoDC=off  ResidualTolerance=1e-9  UseLocalSolver=off  LocalSolverChoice=NE_BACKWARD_EULER_ADVANCER  LocalSolverSampleTime=.001  DoFixedCost=off  MaxNonlinIter=3  MaxModeIter=2  LinearAlgebra=Sparse  DelaysMemoryBudget=1024  AutomaticFiltering=on  FilteringTimeConstant=0.001
  Sugárzott hő a padlótól : fl_lib/Thermal/Thermal Elements/Convective Heat Transfer  area=16 m^2  heat_tr_coeff=5.4 W/(m^2 * K)  Q_specify=off  Q_priority=None  Q=0 J/s  T_specify=off  T_priority=None  T=0 K
  Sunshine : fl_lib/Thermal/Thermal Sources/Ideal Heat Flow Source
  Sunshine1 : fl_lib/Thermal/Thermal Sources/Ideal Heat Flow Source
  Szoba levegője : fl_lib/Thermal/Thermal Elements/Thermal Mass  mass=M_air kg  sp_heat=c_air J/kg/K  T_specify=on  T_priority=High  T=TinIC degC  Q_specify=off  Q_priority=None  Q=0 J/s
  TRef : fl_lib/Thermal/Thermal Elements/Thermal Reference
  TRef1 : fl_lib/Thermal/Thermal Elements/Thermal Reference
  TRef2 : fl_lib/Thermal/Thermal Elements/Thermal Reference
  Heat_convective : PMIOPort  Port=1  Side=Left
  T_in : Outport
  T_wall_out : Outport  Port=2
  Q_wall_out : Outport  Port=3
  Q_conv_in : Outport  Port=4
  Q_le_padlo : Outport  Port=5
  wires:
  T_ext/1 -> S2PS/1
  PS2S1/1 -> Q_wall_out/1
  PS2S3/1 -> Q_conv_in/1
  Padlofutes/1 -> S2PS1/1
  PS2S4/1 -> Q_le_padlo/1
  Falfutes/1 -> S2PS2/1
  MeasTemp/1(T) -> T_wall_out/1
  MeasTemp1/1(Out1) -> T_in/1
  connections:
  Külső oldal - A teljes rétegtervi hőátbocsátási tényező fele/RConn1 -- MeasTemp/LConn1 -- Külső fal/LConn1 -- Belső oldal - A teljes rétegtervi hőátbocsátási tényező másik fele/LConn1
  Külső oldal - A teljes rétegtervi hőátbocsátási tényező fele/LConn1 -- Ideal Heat Flow Sensor/RConn2 -- Ablak/LConn1
  Külső hőmérséklet/RConn2 -- TRef/LConn1
  Solver Configuration/RConn1 -- S2PS/RConn1 -- Külső hőmérséklet/RConn1
  Padló - > levegő/LConn1 -- Sugárzott hő a padlótól/LConn1 -- Padlófűtés / nap/LConn1
  Belső falak/RConn1 -- Sugárzott hő a padlótól/RConn1 -- Sunshine1/LConn1 -- "Fűtött terek közti válaszfalak, mennyezet"/LConn1
  Külső hőmérséklet/LConn1 -- Ideal Heat Flow Sensor/LConn1
  Szoba levegője/LConn1 -- MeasTemp1/LConn1 -- Ablak/RConn1 -- Belső oldal - A teljes rétegtervi hőátbocsátási tényező másik fele/RConn1 -- Ideal Heat Flow Sensor2/RConn2 -- Belső falak/LConn1 -- Padló - > levegő/RConn1
  PS2S1/LConn1 -- Ideal Heat Flow Sensor/RConn1
  Ideal Heat Flow Sensor2/LConn1 -- Heat_convective/RConn1
  Ideal Heat Flow Sensor2/RConn1 -- PS2S3/LConn1
  Sunshine/RConn1 -- S2PS1/RConn1
  Sunshine/RConn2 -- TRef1/LConn1
  PS2S4/LConn1 -- Padlófűtés / nap/RConn1
  Sunshine/LConn1 -- Padlófűtés / nap/RConn2 -- Padló1/LConn1
  Sunshine1/RConn2 -- TRef2/LConn1
  Sunshine1/RConn1 -- S2PS2/RConn1

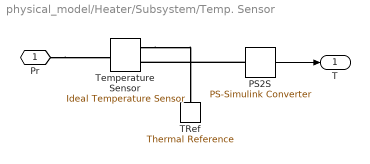
== system physical_model/Heater/Subsystem/Temp. Sensor ==
  PS2S : nesl_utility/PS-Simulink Converter  PhysicalDomain=network_engine_domain  SubClassName=ps_output  LeftPortType=input  RightPortType=output  PseudoPeriodic=off  Frequencies=[]  Unit=degC  AffineConversion=on
  TRef : fl_lib/Thermal/Thermal Elements/Thermal Reference
  Temperature Sensor : fl_lib/Thermal/Thermal Sensors/Ideal Temperature Sensor
  Pr : PMIOPort  Port=1  Side=Left
  T : Outport
  wires:
  PS2S/1 -> T/1
  connections:
  Temperature Sensor/RConn1 -- TRef/LConn1
  PS2S/LConn1 -- Temperature Sensor/RConn2
  Pr/RConn1 -- Temperature Sensor/LConn1

== system physical_model/Heater/Subsystem/Temp. Sensor1 ==
  PS2S : nesl_utility/PS-Simulink Converter  PhysicalDomain=network_engine_domain  SubClassName=ps_output  LeftPortType=input  RightPortType=output  PseudoPeriodic=off  Frequencies=[]  Unit=degC  AffineConversion=on
  TRef : fl_lib/Thermal/Thermal Elements/Thermal Reference
  Temperature Sensor : fl_lib/Thermal/Thermal Sensors/Ideal Temperature Sensor
  Pr : PMIOPort  Port=1  Side=Left
  T : Outport
  wires:
  PS2S/1 -> T/1
  connections:
  Temperature Sensor/RConn1 -- TRef/LConn1
  PS2S/LConn1 -- Temperature Sensor/RConn2
  Pr/RConn1 -- Temperature Sensor/LConn1

== system physical_model/Heater/Subsystem/Temp. Sensor2 ==
  PS2S : nesl_utility/PS-Simulink Converter  PhysicalDomain=network_engine_domain  SubClassName=ps_output  LeftPortType=input  RightPortType=output  PseudoPeriodic=off  Frequencies=[]  Unit=degC  AffineConversion=on
  TRef : fl_lib/Thermal/Thermal Elements/Thermal Reference
  Temperature Sensor : fl_lib/Thermal/Thermal Sensors/Ideal Temperature Sensor
  Pr : PMIOPort  Port=1  Side=Left
  T : Outport
  wires:
  PS2S/1 -> T/1
  connections:
  Temperature Sensor/RConn1 -- TRef/LConn1
  PS2S/LConn1 -- Temperature Sensor/RConn2
  Pr/RConn1 -- Temperature Sensor/LConn1

== system physical_model/House/House Simscape/MeasTemp ==
  PS2S2 : nesl_utility/PS-Simulink Converter  PhysicalDomain=network_engine_domain  SubClassName=ps_output  LeftPortType=input  RightPortType=output  PseudoPeriodic=off  Frequencies=[]  Unit=degC  AffineConversion=on
  TRef4 : fl_lib/Thermal/Thermal Elements/Thermal Reference
  Temperature Sensor1 : fl_lib/Thermal/Thermal Sensors/Ideal Temperature Sensor
  T_meas : PMIOPort  Port=1  Side=Left
  T : Outport
  wires:
  PS2S2/1 -> T/1
  connections:
  Temperature Sensor1/LConn1 -- T_meas/RConn1
  PS2S2/LConn1 -- Temperature Sensor1/RConn2
  Temperature Sensor1/RConn1 -- TRef4/LConn1

== system physical_model/House/House Simscape/MeasTemp1 ==
  PS2S2 : nesl_utility/PS-Simulink Converter  PhysicalDomain=network_engine_domain  SubClassName=ps_output  LeftPortType=input  RightPortType=output  PseudoPeriodic=off  Frequencies=[]  Unit=degC  AffineConversion=on
  TRef4 : fl_lib/Thermal/Thermal Elements/Thermal Reference
  Temperature Sensor1 : fl_lib/Thermal/Thermal Sensors/Ideal Temperature Sensor
  Conn1 : PMIOPort  Port=1  Side=Left
  Out1 : Outport
  wires:
  PS2S2/1 -> Out1/1
  connections:
  Temperature Sensor1/LConn1 -- Conn1/RConn1
  PS2S2/LConn1 -- Temperature Sensor1/RConn2
  Temperature Sensor1/RConn1 -- TRef4/LConn1
